simulink model "PipeGeometry_1"  (Simulink 8.2)
settings: Solver=ode45  StartTime=0.0  StopTime=3600  RelTol=1e-5
libraries: carnot x5
settings Model: Creator=drhf  LastModifiedBy=drhf

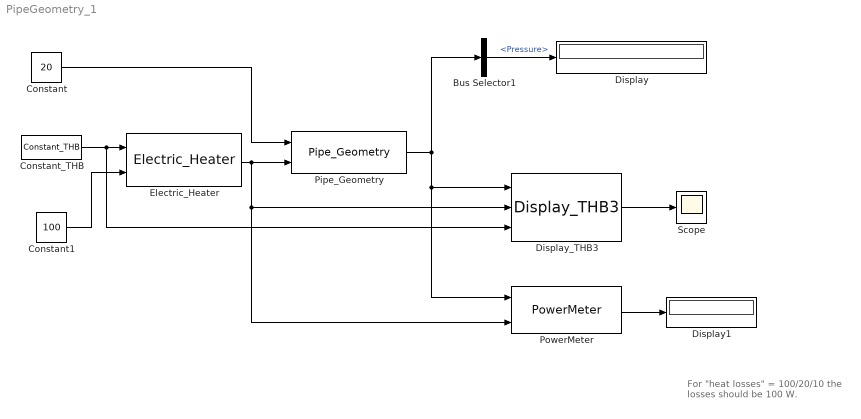
== system PipeGeometry_1 ==
  note: For "heat losses" = 100/20/10
      | the losses should be 100 W.
  Bus Selector1 : BusSelector  OutputSignals=Pressure
  Constant : Constant  Value=20
  Constant1 : Constant  Value=100
  Constant_THB : carnot/Source/Simple/Constant_THB  t=40  mdot=600/3600  p=2e5  mID=Full Pressure Drop with Static Height  fluid=Water  mix=0  dia=10  hgt=0
  Display : Display
      settings: Format=decimal (Stored Integer)
  Display1 : Display
  Display_THB3 : carnot/Outputs/Display_THB3  t=on  m=off  p=off  id=off  mix=off  d=off
  Electric_Heater : carnot/Source/Boiler/Electric_Heater
  Pipe_Geometry : carnot/Hydraulics/Pipe_Geometry  dia=0.02  len=10  hgt=10  uloss=100/20/10  cond=0  cwall=1000  t0=20  rough=0.04*1e-3  nbend=4  nodes=1
  PowerMeter : carnot/Control/PowerMeter
  Scope : Scope
      settings: TimeRange=4000  YMin=39.66951326595616  YMax=40.42277164649369
  wires:
  Constant/1 -> Pipe_Geometry/1
  Pipe_Geometry/1 -> Bus Selector1/1, Display_THB3/1, PowerMeter/1
  Bus Selector1/1 -> Display/1  "<Pressure>"
  Constant_THB/1 -> Display_THB3/3, Electric_Heater/1
  Electric_Heater/1 -> Display_THB3/2, PowerMeter/2, Pipe_Geometry/2
  Constant1/1 -> Electric_Heater/2
  Display_THB3/1 -> Scope/1
  PowerMeter/1 -> Display1/1
